simulink model "multiple_sin"  (R2017a)
settings: Solver=VariableStepAuto  StartTime=0.0  StopTime=T  RelTol=1e-3
values from neighbouring files (symbols this model uses):
  f1 = f    (= 5)    [Time_constant_new.m]    (also in data_generate (PC's conflicted copy 2017-12-16).m; time_constant_testbench.m)
  f2 = f1 * 1.5    (= 7.5)    [Time_constant_new.m]    (also in data_generate (PC's conflicted copy 2017-12-16).m; time_constant_testbench.m)
  f3 = f1 * 1.75    (= 8.75)    [Time_constant_new.m]    (also in data_generate (PC's conflicted copy 2017-12-16).m; time_constant_testbench.m)
  f4 = f1 * 2    (= 10)    [Time_constant_new.m]    (also in data_generate (PC's conflicted copy 2017-12-16).m; time_constant_testbench.m)
  Fs = 1000    [MAR.m]    (also in Time_constant_new.m; corr_multi_sine.m = config(3); csd_damping_sine.m = config(3); csd_fft_testing.m = 100)
  noise_amplitude = 1e-1    (= 0.1)    [MAR.m]    (also in Time_constant_new.m = 1e-05; csd_fft_testing.m; damping_sine.m = config(4); data_generate (PC's conflicted copy 2017-12-16).m = 1e-05)
  ramp_slope = -1    [MAR.m]    (also in Time_constant_new.m; csd_fft_testing.m; damping_sine.m = config(5); data_generate (PC's conflicted copy 2017-12-16).m)
  seed = randi([0 1000],1)    [MAR.m]    (also in TC_iteration.m; Time_constant_new.m; csd_fft_testing.m; damping_sine.m = config(8))
  sin_amplitude1 = 1    [Time_constant_new.m]    (also in data_generate (PC's conflicted copy 2017-12-16).m; time_constant_testbench.m)
  sin_amplitude2 = 0.75    [Time_constant_new.m]    (also in data_generate (PC's conflicted copy 2017-12-16).m; time_constant_testbench.m)
  sin_amplitude3 = 0.5    [Time_constant_new.m]    (also in data_generate (PC's conflicted copy 2017-12-16).m; time_constant_testbench.m)
  sin_amplitude4 = 0.25    [Time_constant_new.m]    (also in data_generate (PC's conflicted copy 2017-12-16).m; time_constant_testbench.m)
libraries: dspsrcs4 x4, simulink x2
settings Model: Creator=ljxia  LastModifiedBy=ljxia

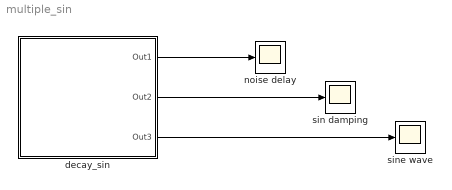
== system multiple_sin ==
  "decay_sin " : Subsystem
  noise delay : Scope
  sin damping : Scope
  sine wave : Scope
  wires:
  "decay_sin "/1(Out1) -> noise delay/1
  "decay_sin "/2(Out2) -> sin damping/1
  "decay_sin "/3(Out3) -> sine wave/1

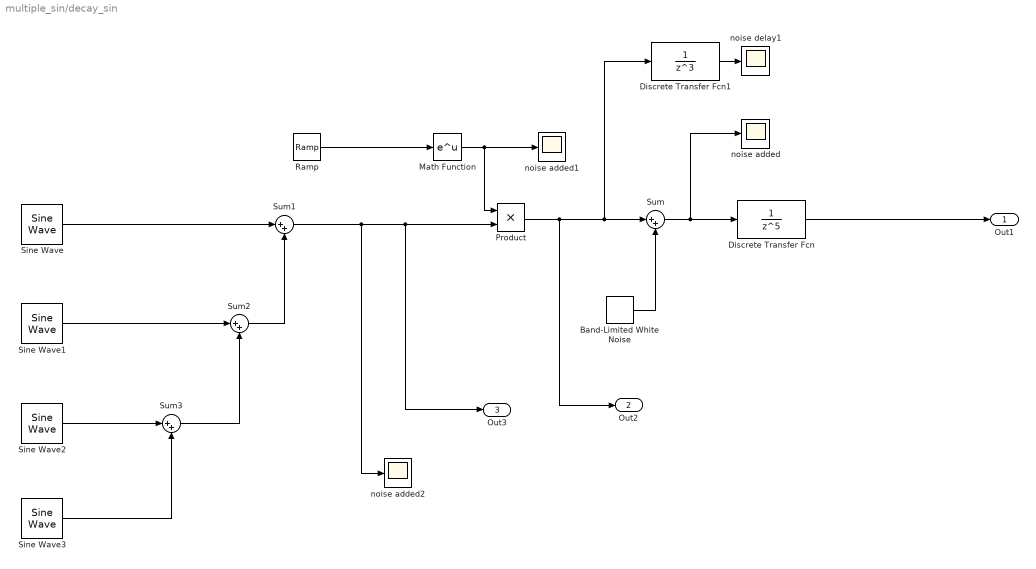
== system multiple_sin/decay_sin  ==
  Band-Limited White Noise : simulink/Sources/Band-Limited White Noise  Cov=[noise_amplitude]  Ts=1/Fs  seed=[seed]
  Discrete Transfer Fcn : DiscreteTransferFcn  Denominator=[1 0 0 0 0 0]
  Discrete Transfer Fcn1 : DiscreteTransferFcn  Denominator=[1 0 0 0]  SampleTime=1/Fs
  Math Function : Math  SaturateOnIntegerOverflow=on
  Product : Product
  Ramp : simulink/Sources/Ramp  slope=ramp_slope  start=0  X0=0
  Sine Wave : dspsrcs4/Sine Wave  Amplitude=sin_amplitude1  Frequency=f1  Phase=0  SampleMode=Discrete  OutComplex=Real  CompMethod=Trigonometric fcn  TableSize=Speed  SampleTime=1/Fs  SamplesPerFrame=1  ResetState=Restart at time zero  OutputFrames=off  dataType=double  wordLen=16  udDataType=sfix(16)  fracBitsMode=Best precision  numFracBits=15  OutDataTypeStr=double  LastOutDataTypeStr=double
  Sine Wave1 : dspsrcs4/Sine Wave  Amplitude=sin_amplitude2  Frequency=f2  Phase=0  SampleMode=Discrete  OutComplex=Real  CompMethod=Trigonometric fcn  TableSize=Speed  SampleTime=1/Fs  SamplesPerFrame=1  ResetState=Restart at time zero  OutputFrames=off  dataType=double  wordLen=16  udDataType=sfix(16)  fracBitsMode=Best precision  numFracBits=15  OutDataTypeStr=double  LastOutDataTypeStr=double
  Sine Wave2 : dspsrcs4/Sine Wave  Amplitude=sin_amplitude3  Frequency=f3  Phase=0  SampleMode=Discrete  OutComplex=Real  CompMethod=Trigonometric fcn  TableSize=Speed  SampleTime=1/Fs  SamplesPerFrame=1  ResetState=Restart at time zero  OutputFrames=off  dataType=double  wordLen=16  udDataType=sfix(16)  fracBitsMode=Best precision  numFracBits=15  OutDataTypeStr=double  LastOutDataTypeStr=double
  Sine Wave3 : dspsrcs4/Sine Wave  Amplitude=sin_amplitude4  Frequency=f4  Phase=0  SampleMode=Discrete  OutComplex=Real  CompMethod=Trigonometric fcn  TableSize=Speed  SampleTime=1/Fs  SamplesPerFrame=1  ResetState=Restart at time zero  OutputFrames=off  dataType=double  wordLen=16  udDataType=sfix(16)  fracBitsMode=Best precision  numFracBits=15  OutDataTypeStr=double  LastOutDataTypeStr=double
  Sum{,1..3} (4 alike) : Sum  Inputs=|++
  noise added : Scope
  noise added1 : Scope
  noise added2 : Scope
  noise delay1 : Scope
  Out1 : Outport
  Out2 : Outport  Port=2
  Out3 : Outport  Port=3
  wires:
  Discrete Transfer Fcn1/1 -> noise delay1/1
  Math Function/1 -> noise added1/1, Product/1
  Product/1 -> Out2/1, Discrete Transfer Fcn1/1, Sum/1
  Sum/1 -> noise added/1, Discrete Transfer Fcn/1
  Ramp/1 -> Math Function/1
  Band-Limited White Noise/1 -> Sum/2
  Discrete Transfer Fcn/1 -> Out1/1
  Sum1/1 -> noise added2/1, Out3/1, Product/2
  Sine Wave/1 -> Sum1/1
  Sine Wave3/1 -> Sum3/2
  Sine Wave2/1 -> Sum3/1
  Sum3/1 -> Sum2/2
  Sine Wave1/1 -> Sum2/1
  Sum2/1 -> Sum1/2
